simulink subsystem "PvtSubSys_VSM_ESS"  (R2020b)
settings: Solver=VariableStepAuto  StartTime=0.0  StopTime=10.0  RelTol=1e-3
values from neighbouring files (symbols this model uses):
  P_VSM_ESS_AccelPed_enable = 1.0    [ESS.sldd]
  P_VSM_ESS_AccPedlPosn_Param = 60.0    [ESS.sldd]
  P_VSM_ESS_ACtiveTime = 5.0    [ESS.sldd]
  P_VSM_ESS_AEBFlag_enable = 1.0    [ESS.sldd]
  P_VSM_ESS_AngleSpdTable_deg : value not decoded    [ESS.sldd]
  P_VSM_ESS_DangerPlausLeft = 0.3    [ESS.sldd]
  P_VSM_ESS_DangerPlausRight = 0.3    [ESS.sldd]
  P_VSM_ESS_DelayTime = 3.0    [ESS.sldd]
  P_VSM_ESS_DoorSts_enable = 1.0    [ESS.sldd]
  P_VSM_ESS_DriveIn : value not decoded    [ESS.sldd]
  P_VSM_ESS_DriveIn_BP : value not decoded    [ESS.sldd]
  P_VSM_ESS_DriverInputdSameDire_delaytime = 1.0    [ESS.sldd]
  P_VSM_ESS_DriverInputTrq_Param : value not decoded    [ESS.sldd]
  P_VSM_ESS_DrvOverTime_Param = 0.2    [ESS.sldd]
  P_VSM_ESS_DrvOverTime_Paramsame = 0.2    [ESS.sldd]
  P_VSM_ESS_DrvSBR_enable = 1.0    [ESS.sldd]
  P_VSM_ESS_ESPActive_enable = 1.0    [ESS.sldd]
  P_VSM_ESS_ESPFuncOffSts_enable = 1.0    [ESS.sldd]
  P_VSM_ESS_FcwDisFlag_enable = 1.0    [ESS.sldd]
  P_VSM_ESS_FcwSw_enable = 1.0    [ESS.sldd]
  P_VSM_ESS_HiLoBeam_enable = 1.0    [ESS.sldd]
  P_VSM_ESS_IPSpeed_kmh : value not decoded    [ESS.sldd]
  P_VSM_ESS_LateralAccel_enable = 1.0    [ESS.sldd]
  P_VSM_ESS_LgtAccelLower_Param = -8.0    [ESS.sldd]
  P_VSM_ESS_LgtAccelUpper_Param = 3.0    [ESS.sldd]
  P_VSM_ESS_MasterCylindBrake = 5.0    [ESS.sldd]
  P_VSM_ESS_MaxLateral_mss : value not decoded    [ESS.sldd]
  P_VSM_ESS_OVERRIDE_SW = 0.0    [ESS.sldd]
  P_VSM_ESS_SafeDistance_m = 1.5    [ESS.sldd]
  P_VSM_ESS_SpdPoint_kmh : value not decoded    [ESS.sldd]
  P_VSM_ESS_SpdTime_s : value not decoded    [ESS.sldd]
  P_VSM_ESS_SteerWheelSpd_BP : value not decoded    [ESS.sldd]
  P_VSM_ESS_SteerWheelSpd_enable = 1.0    [ESS.sldd]
  P_VSM_ESS_SteerWheelSpd_Param : value not decoded    [ESS.sldd]
  P_VSM_ESS_StopA0_Param = 0.2    [ESS.sldd]
  P_VSM_ESS_StopA1_Param = 0.02    [ESS.sldd]
  P_VSM_ESS_StopA1Time_Param = 2.0    [ESS.sldd]
  P_VSM_ESS_TrailerSts_enable = 1.0    [ESS.sldd]
  P_VSM_ESS_VehLgtAccel_enable = 1.0    [ESS.sldd]
  P_VSM_ESS_Vehspeed_enable = 1.0    [ESS.sldd]
  P_VSM_ESS_WiprReq_enable = 1.0    [ESS.sldd]
undefined symbols (not defined in the file or in its folder): P_Global_WheelBase_m
libraries: simulink x104, TrueDurationTime x6
(part 2 of 3)

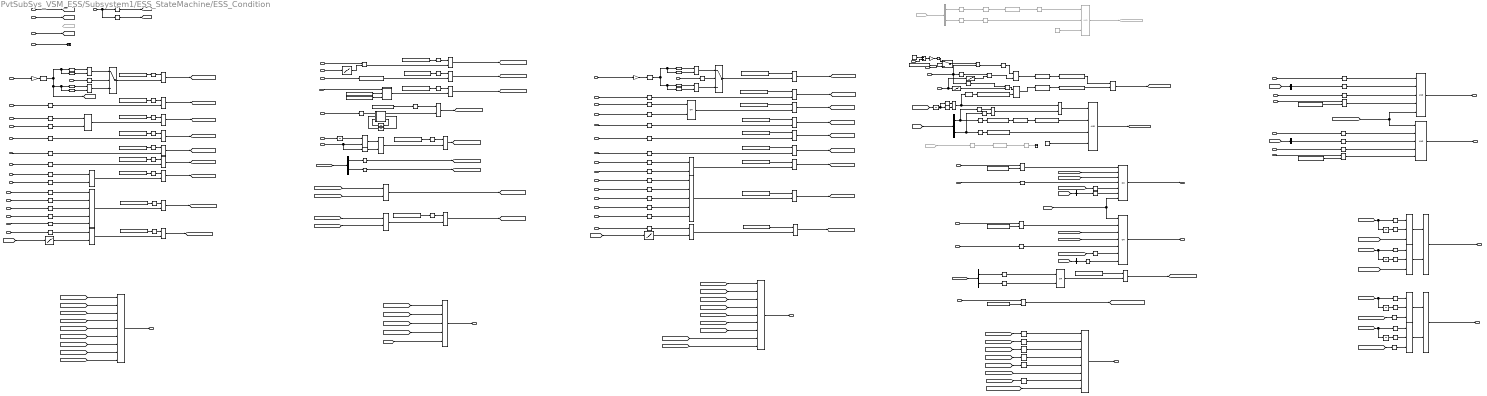
== system PvtSubSys_VSM_ESS/Subsystem1/ESS_StateMachine/ESS_Condition ==
  note: READY2ACYIVE
  note: READY2IDLE
  note: IDLE2READY
  note: PathCondition
  note: EXIT2Ready
  canABSVehicleSpd : Inport
  canESPVDCActive : Inport  Port=2
  canESPPTCActive : Inport  Port=3
  canESPBTCActive : Inport  Port=4
  canABSABSActive : Inport  Port=5
  canEPSEPS_DriverInputTrqValue : Inport  Port=6
  canSASSteerWheelSpd : Inport  Port=7
  canECMAccrPedlPosnDiagc : Inport  Port=8
  canABMLateralAcce : Inport  Port=9
  Torq : Inport  Port=10
  SteerWheelSpdSign : Inport  Port=11
  canBCMWiperSwitchSts : Inport  Port=12
  canBCMHighBeamSts : Inport  Port=13
  canBCMLowBeamSts : Inport  Port=14
  ESPFuncOffSts : Inport  Port=15
  DrvDoorSts : Inport  Port=16
  PassengerDoorSts : Inport  Port=17
  DrvSBR : Inport  Port=18
  canABMLgtAccel : Inport  Port=19
  canESPMSRActive : Inport  Port=20
  canESS_PedSwtReq : Inport  Port=21
  canESP_MasterCylindBrakePress : Inport  Port=22
  TrailerSts : Inport  Port=23
  DangerPlausLeft : Inport  Port=24
  DangerPlausRight : Inport  Port=25
  L_Oncoming_flag : Inport  Port=26
  R_Oncoming_flag : Inport  Port=27
  AEB_Type : Inport  Port=28
  AEBRange : Inport  Port=29
  FCW_Warn : Inport  Port=30
  D_LastPoint : Inport  Port=31
  Target_Line : Inport  Port=32
  ESSState : Inport  Port=33
  AEBTrig : Inport  Port=34
  Dia_inhibit : Inport  Port=35
  steeranglesign : Inport  Port=36
  1-D Lookup Table : Lookup_n-D  NumberOfTableDimensions=1  BreakpointsForDimension1=P_VSM_ESS_IPSpeed_kmh  Table=P_VSM_ESS_MaxLateral_mss  InternalRulePriority=Speed  RndMeth=Simplest  InputSameDT=on
  1-D Lookup Table1 : Lookup_n-D  NumberOfTableDimensions=1  BreakpointsForDimension1=P_VSM_ESS_IPSpeed_kmh  Table=P_VSM_ESS_MaxLateral_mss  InternalRulePriority=Speed  RndMeth=Simplest  InputSameDT=on
  1-D Lookup Table2 : Lookup_n-D  NumberOfTableDimensions=1  BreakpointsForDimension1=P_VSM_ESS_SteerWheelSpd_BP  Table=P_VSM_ESS_SteerWheelSpd_Param  ExtrapMethod=Clip  UseLastTableValue=on  InternalRulePriority=Speed  RndMeth=Simplest  InputSameDT=on
  1-D Lookup Table3 : Lookup_n-D  NumberOfTableDimensions=1  BreakpointsForDimension1=P_VSM_ESS_DriveIn_BP  Table=P_VSM_ESS_DriveIn  InternalRulePriority=Speed  RndMeth=Simplest  InputSameDT=on
  1-D Lookup Table4 : Lookup_n-D  NumberOfTableDimensions=1  BreakpointsForDimension1=P_VSM_ESS_DriveIn_BP  Table=P_VSM_ESS_DriverInputTrq_Param  InternalRulePriority=Speed  RndMeth=Simplest  InputSameDT=on
  ACTIVE2IDLE : Logic  Operator=OR  Inputs=8  AllPortsSameDT=off  OutDataTypeStr=boolean
  Abs{,1,3,16..18} (6 alike) : Abs
  Abs19 : Abs  Commented=on
  Abs2 : Abs  Commented=on
  Add : Sum  Inputs=-+
  Bias4 : Bias  Bias=1.3
  Bias7 : Bias  Bias=1.3
  Bus Selector1 : BusSelector  OutputSignals=ESSLineLValid
  Bus Selector13 : BusSelector  OutputSignals=AEB_PedTrig,AEB_VehTrig
  Bus Selector2 : BusSelector  OutputSignals=AEB_PedTrig,AEB_VehTrig
  Bus Selector20 : BusSelector  OutputSignals=ESSLineA1,ESSLineA0
  Bus Selector21 : BusSelector  Commented=on  OutputSignals=ESSLineA1,ESSLineA0
  Bus Selector3 : BusSelector  OutputSignals=ESSLineLValid
  Bus Selector4 : BusSelector  OutputSignals=ESSLineRValid
  Bus Selector5 : BusSelector  OutputSignals=ESSLineRValid
  Compare To Constant{,11,13,15} (4 alike) : simulink/Logic and Bit Operations/Compare To Constant  relop===  const=2  OutDataTypeStr=boolean
  Compare To Constant1 : simulink/Logic and Bit Operations/Compare To Constant  relop=>=  const=P_VSM_ESS_DrvOverTime_Param  OutDataTypeStr=boolean
  Compare To Constant10 : simulink/Logic and Bit Operations/Compare To Constant  relop===  const=4  OutDataTypeStr=boolean
  Compare To Constant{3,8..9,18,20..32,113,181,184..185,193,195,200..201,214..215,220..224,237} (33 alike) : simulink/Logic and Bit Operations/Compare To Constant  relop===  const=0  OutDataTypeStr=boolean
  Compare To Constant12 : simulink/Logic and Bit Operations/Compare To Constant  relop===  const=5  OutDataTypeStr=boolean
  Compare To Constant14 : simulink/Logic and Bit Operations/Compare To Constant  relop===  const=4  OutDataTypeStr=boolean
  Compare To Constant16 : simulink/Logic and Bit Operations/Compare To Constant  relop===  const=5  OutDataTypeStr=boolean
  Compare To Constant166 : simulink/Logic and Bit Operations/Compare To Constant  relop=>=  const=50  OutDataTypeStr=boolean
  Compare To Constant17 : simulink/Logic and Bit Operations/Compare To Constant  relop=>  const=0  OutDataTypeStr=boolean
  Compare To Constant176 : simulink/Logic and Bit Operations/Compare To Constant  relop=<=  const=100  OutDataTypeStr=boolean
  Compare To Constant179 : simulink/Logic and Bit Operations/Compare To Constant  relop=<=  const=45  OutDataTypeStr=boolean
  Compare To Constant180 : simulink/Logic and Bit Operations/Compare To Constant  relop=>=  const=105  OutDataTypeStr=boolean
  Compare To Constant{6..7,183,188..190,194,196..197,202,205,217..219,226..228,232,235,239..240} (21 alike) : simulink/Logic and Bit Operations/Compare To Constant  relop===  const=1  OutDataTypeStr=boolean
  Compare To Constant19 : simulink/Logic and Bit Operations/Compare To Constant  relop===  const=4  OutDataTypeStr=boolean
  Compare To Constant198 : simulink/Logic and Bit Operations/Compare To Constant  relop=<  const=3  OutDataTypeStr=boolean
  Compare To Constant199 : simulink/Logic and Bit Operations/Compare To Constant  relop===  const=3  OutDataTypeStr=boolean
  Compare To Constant2 : simulink/Logic and Bit Operations/Compare To Constant  relop=>=  const=P_VSM_ESS_StopA1Time_Param  OutDataTypeStr=boolean
  Compare To Constant207 : simulink/Logic and Bit Operations/Compare To Constant  relop=<  const=P_VSM_ESS_AccPedlPosn_Param  OutDataTypeStr=boolean
  Compare To Constant211 : simulink/Logic and Bit Operations/Compare To Constant  relop=<=  const=P_VSM_ESS_StopA1_Param  OutDataTypeStr=boolean
  Compare To Constant212 : simulink/Logic and Bit Operations/Compare To Constant  relop=>  const=0  OutDataTypeStr=boolean
  Compare To Constant216 : simulink/Logic and Bit Operations/Compare To Constant  relop=<=  const=P_VSM_ESS_StopA0_Param  OutDataTypeStr=boolean
  Compare To Constant229 : simulink/Logic and Bit Operations/Compare To Constant  Commented=on  relop=<=  const=0.015  OutDataTypeStr=boolean
  Compare To Constant230 : simulink/Logic and Bit Operations/Compare To Constant  relop=>=  const=50  OutDataTypeStr=boolean
  Compare To Constant231 : simulink/Logic and Bit Operations/Compare To Constant  relop=<=  const=85  OutDataTypeStr=boolean
  Compare To Constant233 : simulink/Logic and Bit Operations/Compare To Constant  relop=<=  const=45  OutDataTypeStr=boolean
  Compare To Constant234 : simulink/Logic and Bit Operations/Compare To Constant  relop=>=  const=90  OutDataTypeStr=boolean
  Compare To Constant236 : simulink/Logic and Bit Operations/Compare To Constant  Commented=on  relop=<=  const=0.2  OutDataTypeStr=boolean
  Compare To Constant33 : simulink/Logic and Bit Operations/Compare To Constant  relop===  const=5  OutDataTypeStr=boolean
  Compare To Constant34 : simulink/Logic and Bit Operations/Compare To Constant  relop=~=  const=0  OutDataTypeStr=boolean
  Compare To Constant35 : simulink/Logic and Bit Operations/Compare To Constant  relop=~=  const=0  OutDataTypeStr=boolean
  Compare To Constant36 : simulink/Logic and Bit Operations/Compare To Constant  relop===  const=3  OutDataTypeStr=boolean
  Compare To Constant37 : simulink/Logic and Bit Operations/Compare To Constant  relop=>=  const=P_VSM_ESS_DriverInputdSameDire_delaytime  OutDataTypeStr=boolean
  Compare To Constant38 : simulink/Logic and Bit Operations/Compare To Constant  relop=>=  const=P_VSM_ESS_DrvOverTime_Paramsame  OutDataTypeStr=boolean
  Compare To Constant4 : simulink/Logic and Bit Operations/Compare To Constant  Commented=on  relop=>=  const=2  OutDataTypeStr=boolean
  Compare To Constant5 : simulink/Logic and Bit Operations/Compare To Constant  Commented=on  relop=>=  const=5  OutDataTypeStr=boolean
  Compare To Zero{,1..5} (6 alike) : simulink/Logic and Bit Operations/Compare To Zero  relop===  OutDataTypeStr=boolean
  Compare To Zero6 : simulink/Logic and Bit Operations/Compare To Zero  relop=<  OutDataTypeStr=boolean
  Compare To Zero7 : simulink/Logic and Bit Operations/Compare To Zero  Commented=on  relop===  OutDataTypeStr=boolean
  Constant : Constant  Value=P_VSM_ESS_DangerPlausLeft
  Constant1 : Constant  Value=P_VSM_ESS_FcwSw_enable
  Constant11 : Constant  OutDataTypeStr=boolean
  Constant12 : Constant  Commented=on  OutDataTypeStr=boolean
  Constant2 : Constant  Value=P_VSM_ESS_MasterCylindBrake
  Constant3 : Constant  Value=P_VSM_ESS_OVERRIDE_SW
  Constant4 : Constant  Value=P_VSM_ESS_DangerPlausRight
  Constant5 : Constant  Value=0.5
  Constant6 : Constant  Value=P_VSM_ESS_DangerPlausLeft
  Constant7 : Constant  Value=P_VSM_ESS_DangerPlausRight
  DangerPlausLeft_1 : InportShadow  Port=24
  DangerPlausRight_1 : InportShadow  Port=25
  DrvDoorSts_1 : InportShadow  Port=16
  DrvSBR_1 : InportShadow  Port=18
  ESPFuncOffSts_1 : InportShadow  Port=15
  ESS_AEBFlag : Logic  AllPortsSameDT=off  OutDataTypeStr=boolean
  ESS_AEBFlag1 : Logic  AllPortsSameDT=off  OutDataTypeStr=boolean
  ESS_AEBFlag2 : Logic  AllPortsSameDT=off  OutDataTypeStr=boolean
  ESS_AEBFlag3 : Logic  Operator=OR  AllPortsSameDT=off  OutDataTypeStr=boolean
  ESS_AEBFlag4 : Logic  Operator=OR  AllPortsSameDT=off  OutDataTypeStr=boolean
  ESS_AEBFlag5 : Logic  Operator=OR  AllPortsSameDT=off  OutDataTypeStr=boolean
  From314 : From  Commented=on  GotoTag=Target_Line
  From316 : From  Commented=on  GotoTag=FCWObjExist
  Gain : Gain  Gain=-2
  Gain15 : Gain  Gain=1.03
  Gain16 : Gain  Gain=1.03
  Goto169 : Goto  Commented=on  GotoTag=ESS_R_Acomp_Active2Ready
  Goto3 : Goto  Commented=on  GotoTag=FCWObjExist
  IDLE2READY : Logic  Inputs=9  AllPortsSameDT=off  OutDataTypeStr=boolean
  L_Oncoming_flag_1 : InportShadow  Port=26
  Logical Operator{,3,6,8..18,28,32,64,103,111,114,128} (21 alike) : Logic  Operator=OR  AllPortsSameDT=off  OutDataTypeStr=boolean
  Logical Operator{1..2,4..5} (4 alike) : Logic  Inputs=3  AllPortsSameDT=off  OutDataTypeStr=boolean
  Logical Operator104 : Logic  Operator=OR  Inputs=7  AllPortsSameDT=off  OutDataTypeStr=boolean
  Logical Operator{7,19..27,29..31,108,110,112..113,127} (18 alike) : Logic  AllPortsSameDT=off  OutDataTypeStr=boolean
  Logical Operator109 : Logic  Operator=OR  Inputs=7  AllPortsSameDT=off  OutDataTypeStr=boolean
  Logical Operator123 : Logic  Inputs=5  AllPortsSameDT=off  OutDataTypeStr=boolean
  Logical Operator125 : Logic  Operator=OR  Inputs=5  AllPortsSameDT=off  OutDataTypeStr=boolean
  Logical Operator45 : Logic  Inputs=5  AllPortsSameDT=off  OutDataTypeStr=boolean
  Logical Operator68 : Logic  Inputs=4  AllPortsSameDT=off  OutDataTypeStr=boolean
  Logical Operator78 : Logic  Inputs=5  AllPortsSameDT=off  OutDataTypeStr=boolean
  Logical Operator81 : Logic  Commented=on  Inputs=3  AllPortsSameDT=off  OutDataTypeStr=boolean
  MATLAB Function : MATLAB Function  TreatAsAtomicUnit=on
  MATLAB Function1 : MATLAB Function  TreatAsAtomicUnit=on
  PassengerDoorSts_1 : InportShadow  Port=17
  Product7 : Product
  READY2ACTIVE : Logic  Inputs=5  AllPortsSameDT=off  OutDataTypeStr=boolean
  READY2IDLE : Logic  Operator=OR  Inputs=9  AllPortsSameDT=off  OutDataTypeStr=boolean
  R_Oncoming_flag_1 : InportShadow  Port=27
  Relational Operator : RelationalOperator  Operator=<=  OutDataTypeStr=boolean  RndMeth=Simplest
  Relational Operator1 : RelationalOperator  Operator=<=  OutDataTypeStr=boolean  RndMeth=Simplest
  Relational Operator13 : RelationalOperator  OutDataTypeStr=boolean  RndMeth=Nearest
  Relational Operator{2..3,5..9} (7 alike) : RelationalOperator  Operator=>  OutDataTypeStr=boolean  RndMeth=Simplest
  Relational Operator4 : RelationalOperator  Operator=<  OutDataTypeStr=boolean  RndMeth=Simplest
  Sign : Signum
  Signal Copy{1..6} (6 alike) : SignalConversion  OverrideOpt=off
  SteerWheelSpdSign_1 : InportShadow  Port=11
  Switch : Switch  Criteria=u2 > Threshold
  Switch10 : Switch  Criteria=u2 ~= 0
  Switch11 : Switch  Criteria=u2 ~= 0
  Terminator : Terminator
  Terminator10 : Terminator
  TrailerSts_1 : InportShadow  Port=23
  TrueDurationTime{,1,4..5} (4 alike) : TrueDurationTime/TrueDurationTime  TCycle=0.02
  TrueDurationTime2 : TrueDurationTime/TrueDurationTime  Commented=on  TCycle=0.02
  TrueDurationTime3 : TrueDurationTime/TrueDurationTime  Commented=on  TCycle=0.02
  Unit Delay{,1..7} (8 alike) : UnitDelay  SampleTime=-1  HasFrameUpgradeWarning=on
  canABMLateralAcce_1 : InportShadow  Port=9
  canABSABSActive_1 : InportShadow  Port=5
  canABSVehicleSpd1 : InportShadow
  canABSVehicleSpd_1 : InportShadow
  canABSVehicleSpd_2 : InportShadow
  canBCMHighBeamSts_1 : InportShadow  Port=13
  canBCMLowBeamSts_1 : InportShadow  Port=14
  canBCMWiperSwitchSts_1 : InportShadow  Port=12
  canESPBTCActive_1 : InportShadow  Port=4
  canESPMSRActive_1 : InportShadow  Port=20
  canESPPTCActive_1 : InportShadow  Port=3
  canESPVDCActive_1 : InportShadow  Port=2
  canESS_PedSwtReq_1 : InportShadow  Port=21
  param_1 : Constant  Value=P_VSM_ESS_Vehspeed_enable
  param_10 : Constant  Value=P_VSM_ESS_SteerWheelSpd_enable
  param_11 : Constant  Value=P_VSM_ESS_AccelPed_enable
  param_12 : Constant  Value=P_VSM_ESS_VehLgtAccel_enable
  param_13 : Constant  Value=P_VSM_ESS_FcwDisFlag_enable
  param_14 : Constant  Value=P_VSM_ESS_AEBFlag_enable
  param_15 : Constant  Value=P_VSM_ESS_ESPFuncOffSts_enable
  param_16 : Constant  Value=P_VSM_ESS_DoorSts_enable
  param_17 : Constant  Value=P_VSM_ESS_DrvSBR_enable
  param_18 : Constant  Value=P_VSM_ESS_TrailerSts_enable
  param_19 : Constant  Value=P_VSM_ESS_WiprReq_enable
  param_2 : Constant  Value=P_VSM_ESS_ESPFuncOffSts_enable
  param_20 : Constant  Value=P_VSM_ESS_HiLoBeam_enable
  param_21 : Constant  Value=P_VSM_ESS_ESPActive_enable
  param_22 : Constant  Value=P_VSM_ESS_LateralAccel_enable
  param_23 : Constant  Value=P_VSM_ESS_AEBFlag_enable
  param_24 : Constant  Value=P_VSM_ESS_LgtAccelUpper_Param
  param_25 : Constant  Value=P_VSM_ESS_LgtAccelLower_Param
  param_3 : Constant  Value=P_VSM_ESS_DoorSts_enable
  param_4 : Constant  Value=P_VSM_ESS_DrvSBR_enable
  param_5 : Constant  Value=P_VSM_ESS_TrailerSts_enable
  param_52 : Constant  Value=P_VSM_ESS_Vehspeed_enable
  param_6 : Constant  Value=P_VSM_ESS_WiprReq_enable
  param_7 : Constant  Value=P_VSM_ESS_HiLoBeam_enable
  param_8 : Constant  Value=P_VSM_ESS_ESPActive_enable
  param_9 : Constant  Value=P_VSM_ESS_LateralAccel_enable
  ESSDataClct_DriverSteerESSExit : Outport
  ESSDataClct_OverrideESSExit : Outport  Port=2
  ESS_IDLE2READY : Outport  Port=3
  ESS_READY2ACTIVE : Outport  Port=4
  ESS_READY2IDLE : Outport  Port=5
  ESS_ACTIVE2IDLE : Outport  Port=6
  ESS_L_Active2Ready : Outport  Port=7
  ESS_R_Active2Ready : Outport  Port=8
  ESS_Left_Ready2Active : Outport  Port=9
  ESS_Right_Ready2Active : Outport  Port=10
  wires:
  Abs3/1 -> Relational Operator9/1
  1-D Lookup Table4/1 -> Relational Operator9/2
  Logical Operator32/1 -> [ESS_DrvOver_Active2Ready]  "VSM_ESS_DrvOver_Active2Ready"
  Compare To Constant38/1 -> Logical Operator32/2  "VSM_ESS_DrvOver_Active2Ready_SamDirc"
  TrueDurationTime5/1 -> Compare To Constant38/1
  Logical Operator31/1 -> TrueDurationTime5/1
  Relational Operator8/1 -> Logical Operator31/1
  Compare To Constant37/1 -> Logical Operator31/2
  TrueDurationTime4/1 -> Compare To Constant37/1
  1-D Lookup Table3/1 -> Relational Operator8/2
  Abs/1 -> Relational Operator8/1
  canABSVehicleSpd_2/1 -> 1-D Lookup Table3/1, 1-D Lookup Table4/1
  Sign/1 -> Switch/1
  1-D Lookup Table2/1 -> Relational Operator7/2
  canABSVehicleSpd1/1 -> 1-D Lookup Table2/1
  [Dia_Out] -> Logical Operator104/1, Logical Operator109/7
  [Dia_In] -> READY2ACTIVE/5
  Compare To Constant36/1 -> [Dia_Out]
  Compare To Constant3/1 -> [Dia_In]
  Dia_inhibit/1 -> Compare To Constant3/1, Compare To Constant36/1
  param_25/1 -> MATLAB Function1/3(lower)
  param_24/1 -> MATLAB Function1/2(uper)
  DangerPlausRight_1/1 -> Relational Operator1/1
  Signal Copy5/1 -> ACTIVE2IDLE/5  "VSM_ESS_DrvSBR_ACTIVE2IDLE"
  Compare To Constant16/1 -> Logical Operator5/2
  Compare To Constant211/1 -> TrueDurationTime1/1
  Logical Operator9/1 -> [Con_DoorSts_Idle2Ready_ESS]  "VSM_ESS_DoorSts_IDLE2READY"
  Compare To Constant216/1 -> Logical Operator68/3  "VSM_ESS_LineA0_Active2Ready"
  Logical Operator104/1 -> ESS_R_Active2Ready/1  "VSM_ESS_R_Active2Ready"
  canSASSteerWheelSpd/1 -> Relational Operator7/1
  [Con_HiLoBeam_Ready2Idle_ESS] -> READY2IDLE/7
  Unit Delay5/1 -> Compare To Constant16/1
  [Con_AccelPedl_Ready2Active_ESS] -> READY2ACTIVE/3
  [Con_AEBFlag_Ready2Active_ESS] -> READY2ACTIVE/2
  [Con_FcwFlag_Ready2Active_ESS] -> READY2ACTIVE/1
  Bias4/1 -> Compare To Constant230/1, Compare To Constant231/1, [IP_Speed], Compare To Constant176/1, Compare To Constant166/1
  [Con_HiLoBeam_Idle2Ready_ESS] -> IDLE2READY/7
  Logical Operator1/1 -> Logical Operator3/1
  canESPMSRActive/1 -> Compare To Constant221/1
  [Con_WiprReq_Ready2Idle_ESS] -> READY2IDLE/6
  Signal Copy3/1 -> ACTIVE2IDLE/4  "VSM_ESS_DoorSts_ACTIVE2IDLE"
  Compare To Constant179/1 -> Logical Operator128/1
  DrvDoorSts/1 -> Compare To Constant184/1
  [Con_DoorSts_Idle2Ready_ESS] -> IDLE2READY/3
  Compare To Constant231/1 -> Logical Operator127/2
  [Con_VehLgtAccel_Ready2Active_ESS] -> READY2ACTIVE/4
  Bus Selector4/1 -> Compare To Constant196/1  "<ESSLineRValid>"
  canABSABSActive_1/1 -> Compare To Constant227/1
  Compare To Zero/1 -> Logical Operator45/3  "VSM_ESS_LeftOncoming_Ready2Active"
  Compare To Constant226/1 -> Logical Operator125/3
  Logical Operator108/1 -> TrueDurationTime/1
  ESS_AEBFlag1/1 -> [Con_FcwFlag_Ready2Active_ESS]  "VSM_ESS_FcwFlag_READY2ACTIVE"
  SteerWheelSpdSign_1/1 -> Compare To Constant217/1
  Compare To Constant180/1 -> Logical Operator128/2
  [Con_ESPFuncOffSts_Ready2Idle_ESS] -> READY2IDLE/2
  Compare To Constant227/1 -> Logical Operator125/5
  [Con_DrvSBR_Idle2Ready_ESS] -> IDLE2READY/4
  Signal Copy1/1 -> ACTIVE2IDLE/2  "VSM_ESS_LateralAccel_ACTIVE2IDLE"
  [Con_VehicleSpeed_Idle2Ready_ESS] -> IDLE2READY/1
  Bus Selector13/1 -> Compare To Constant214/1  "<AEB_PedTrig>"
  Abs17/1 -> Relational Operator5/1
  [Target_Line] -> Bus Selector5/1
  canESPPTCActive/1 -> Compare To Constant223/1
  R_Oncoming_flag_1/1 -> Compare To Zero3/1
  [Con_TrailerSts_Idle2Ready_ESS] -> IDLE2READY/5
  canESPBTCActive/1 -> Compare To Constant224/1
  [Target_Line] -> Bus Selector1/1
  [Con_TrailerSts_Ready2Idle_ESS] -> READY2IDLE/5
  Logical Operator6/1 -> ESSDataClct_OverrideESSExit/1  "ESSDataClct_OverrideESSExit"
  Compare To Zero4/1 -> Logical Operator4/3
  [Con_VehicleSpeed_Ready2Idle_ESS] -> READY2IDLE/1
  canESPVDCActive/1 -> Compare To Constant222/1
  [Con_ABMLateralAcce_Idle2Ready_ESS] -> IDLE2READY/9
  Logical Operator18/1 -> [Con_VehLgtAccel_Ready2Active_ESS]  "VSM_ESS_VehLgtAccel_READY2ACTIVE"
  Compare To Constant219/1 -> Logical Operator125/2
  Constant11/1 -> Logical Operator68/4
  Bias7/1 -> Compare To Constant233/1, Compare To Constant234/1, Compare To Constant180/1, Compare To Constant179/1
  Compare To Constant166/1 -> Logical Operator110/1
  [ESS_Acomp_Active2Ready] -> Logical Operator104/3
  DrvSBR_1/1 -> Compare To Constant194/1
  ESS_AEBFlag5/1 -> [Con_AEBFlag_Ready2Active_ESS]  "VSM_ESS_AEBFlag_READY2ACTIVE"
  PassengerDoorSts/1 -> Compare To Constant185/1
  PassengerDoorSts_1/1 -> Compare To Constant189/1
  Logical Operator21/1 -> [Con_DrvSBR_Ready2Idle_ESS]  "VSM_ESS_DrvSBR_READY2IDLE"
  [Con_DrvSBR_Ready2Idle_ESS] -> READY2IDLE/4
  Signal Copy2/1 -> ACTIVE2IDLE/3  "VSM_ESS_ESPFuncOffSts_ACTIVE2IDLE"
  ESPFuncOffSts/1 -> Compare To Constant181/1
  [Con_WiprReq_Idle2Ready_ESS] -> IDLE2READY/6
  Compare To Constant190/1 -> Logical Operator45/2  "VSM_ESS_LineLValid_Ready2Active"
  Logical Operator127/1 -> Switch10/1
  canABMLgtAccel/1 -> MATLAB Function1/1(LgAcc)
  IDLE2READY/1 -> ESS_IDLE2READY/1
  Compare To Constant237/1 -> Logical Operator45/1  "VSM_ESS_L_SteerWheelSpdSign_Ready2Active"
  Logical Operator7/1 -> [Con_VehicleSpeed_Ready2Idle_ESS]  "VSM_ESS_VehicleSpd_READY2IDLE"
  Logical Operator64/1 -> [Con_VehicleSpeed_Idle2Ready_ESS]  "VSM_ESS_VehicleSpd_IDLE2READY"
  Bus Selector13/2 -> Compare To Constant215/1  "<AEB_VehTrig>"
  [Con_ESPFuncOffSts_Idle2Ready_ESS] -> IDLE2READY/2
  DrvSBR/1 -> Compare To Constant193/1
  ESPFuncOffSts_1/1 -> Compare To Constant183/1
  canESPBTCActive_1/1 -> Compare To Constant228/1
  canBCMHighBeamSts/1 -> Compare To Constant200/1
  TrueDurationTime1/1 -> Compare To Constant2/1
  Abs19/1 -> Compare To Constant229/1
  Logical Operator78/1 -> ESS_Right_Ready2Active/1
  Compare To Constant189/1 -> Logical Operator103/2
  L_Oncoming_flag/1 -> Compare To Constant239/1
  AEBRange/1 -> Unit Delay/1
  Compare To Constant215/1 -> [Con_AEBVehFlag_Ready2Active_ESS]
  TrailerSts_1/1 -> Compare To Constant197/1
  Logical Operator26/1 -> [Con_ABMLateralAcce_Ready2Idle_ESS]  "VSM_ESS_LateralAccel_READY2IDLE"
  [ESSState] -> Unit Delay1/1, Compare To Constant/1
  Compare To Constant240/1 -> Logical Operator104/5  "VSM_ESS_R_Oncoming_Active2Ready"
  DangerPlausLeft/1 -> Relational Operator2/1
  Logical Operator15/1 -> [Con_ABMLateralAcce_Idle2Ready_ESS]  "VSM_ESS_LateralAccel_IDLE2READY"
  Logical Operator11/1 -> [Con_TrailerSts_Idle2Ready_ESS]  "VSM_ESS_TrailerSts_IDLE2READY"
  Compare To Constant222/1 -> Logical Operator123/3
  D_LastPoint/1 -> Compare To Constant17/1, Relational Operator13/2
  Compare To Constant13/1 -> Logical Operator4/1
  Compare To Constant11/1 -> Logical Operator2/1
  Abs16/1 -> Relational Operator4/1
  READY2ACTIVE/1 -> ESS_READY2ACTIVE/1
  [Con_AEBVehFlag_Ready2Active_ESS] -> ESS_AEBFlag/1  "VSM_ESS_AEBVehFlag_Ready2Active"
  Logical Operator25/1 -> [Con_ESPActive_Ready2Idle_ESS]  "VSM_ESS_ESPActive_READY2IDLE"
  ESS_AEBFlag2/1 -> ESS_AEBFlag4/2
  DrvDoorSts_1/1 -> Compare To Constant188/1
  Compare To Constant196/1 -> Logical Operator78/3  "VSM_ESS_LineRValid_Ready2Active"
  canABMLateralAcce/1 -> Abs16/1
  Logical Operator20/1 -> [Con_DoorSts_Ready2Idle_ESS]  "VSM_ESS_DoorSts_READY2IDLE"
  Unit Delay4/1 -> Compare To Constant14/1
  Logical Operator109/1 -> ESS_L_Active2Ready/1  "VSM_ESS_L_Active2Ready"
  Compare To Constant4/1 -> Logical Operator81/1  "VSM_ESS_LineRA1_Active2Ready"
  Bus Selector21/2 -> Abs2/1  "<ESSLineA0>"
  Unit Delay2/1 -> Compare To Constant12/1
  Compare To Constant202/1 -> Logical Operator114/1
  [ESS_DrvOver_Active2Ready] -> Logical Operator104/4
  Relational Operator1/1 -> Logical Operator78/5  "VSM_ESS_DangerPlausRight_Ready2Active"
  Logical Operator68/1 -> [ESS_Acomp_Active2Ready]
  [AEBTrig] -> Bus Selector13/1
  Logical Operator16/1 -> [Con_SteerWheelSpd_Ready2Active_ESS]  "VSM_ESS_SteerWheelSpd_READY2ACTIVE"
  Compare To Constant239/1 -> Logical Operator109/4  "VSM_ESS_L_Oncoming_Active2Ready"
  Relational Operator9/1 -> Logical Operator108/2
  Relational Operator3/1 -> Logical Operator104/2  "VSM_ESS_DPC_R_Active2Ready"
  [Target_Line] -> Bus Selector4/1
  canESS_PedSwtReq_1/1 -> Compare To Constant232/1
  Compare To Zero1/1 -> Logical Operator109/5
  Logical Operator128/1 -> Switch11/3
  [ESSState] -> Unit Delay4/1, Compare To Constant13/1
  L_Oncoming_flag_1/1 -> Compare To Zero/1
  Logical Operator14/1 -> [Con_ESPActive_Idle2Ready_ESS]  "VSM_ESS_ESPActive_IDLE2READY"
  FCW_Warn/1 -> Compare To Constant212/1
  Logical Operator81/1 -> Goto169/1
  Compare To Constant15/1 -> Logical Operator5/1
  Compare To Constant184/1 -> Logical Operator113/1
  AEB_Type/1 -> Terminator/1
  Logical Operator17/1 -> [Con_AccelPedl_Ready2Active_ESS]  "VSM_ESS_AccelPed_READY2ACTIVE"
  Abs2/1 -> Compare To Constant236/1
  Compare To Constant200/1 -> Logical Operator112/1
  Compare To Constant217/1 -> Logical Operator78/2  "VSM_ESS_R_SteerWheelSpdSign_Ready2Active"
  canBCMLowBeamSts/1 -> Compare To Constant201/1
  Compare To Constant5/1 -> Terminator10/1
  Gain15/1 -> Bias4/1
  Compare To Constant223/1 -> Logical Operator123/4
  Compare To Constant188/1 -> Logical Operator103/1
  canBCMLowBeamSts_1/1 -> Compare To Constant205/1
  canABSABSActive/1 -> Compare To Constant220/1
  canEPSEPS_DriverInputTrqValue/1 -> Product7/2, Abs3/1, Abs/1
  Logical Operator23/1 -> [Con_WiprReq_Ready2Idle_ESS]  "VSM_ESS_WiprReq_READY2IDLE"
  Gain16/1 -> Bias7/1
  Product7/1 -> Compare To Zero6/1
  [ESS_DrvOver_Active2Ready] -> Logical Operator2/3
  Logical Operator45/1 -> ESS_Left_Ready2Active/1
  canABMLateralAcce_1/1 -> Abs17/1
  [Con_AEBTrigFlag_Active2Idle_ESS] -> ACTIVE2IDLE/6
  Bus Selector21/1 -> Abs19/1  "<ESSLineA1>"
  Compare To Constant185/1 -> Logical Operator113/2
  Compare To Constant236/1 -> Logical Operator81/2  "VSM_ESS_LineRA0_Active2Ready"
  Compare To Constant1/1 -> Logical Operator32/1  "VSM_ESS_DrvOver_Active2Ready_DiffDirc"
  Bus Selector20/1 -> Compare To Constant34/1, Abs18/1  "<ESSLineA1>"
  Compare To Constant235/1 -> Switch11/2
  Abs18/1 -> Compare To Constant211/1
  [Con_AEBVruFlag_Ready2Active_ESS] -> ESS_AEBFlag/2  "VSM_ESS_AEBVruFlag_Ready2Active"
  TrailerSts/1 -> Compare To Constant195/1
  Compare To Constant234/1 -> Logical Operator111/2
  canESPVDCActive_1/1 -> Compare To Constant219/1
  canABSVehicleSpd_1/1 -> Gain16/1
  Compare To Constant/1 -> Logical Operator1/1
  [ESS_Acomp_Active2Ready] -> Logical Operator109/2
  [Con_ESPActive_Idle2Ready_ESS] -> IDLE2READY/8
  Compare To Constant233/1 -> Logical Operator111/1
  Bus Selector2/1 -> Compare To Constant6/1  "<AEB_PedTrig>"
  Compare To Constant232/1 -> Switch10/2
  Logical Operator24/1 -> [Con_HiLoBeam_Ready2Idle_ESS]  "VSM_ESS_HiLoBeam_READY2IDLE"
  [ESS_DrvOver_Active2Ready] -> Logical Operator109/3
  [Target_Line] -> Bus Selector20/1
  Bus Selector1/1 -> Compare To Constant190/1  "<ESSLineLValid>"
  Bus Selector2/2 -> Compare To Constant7/1  "<AEB_VehTrig>"
  DangerPlausRight/1 -> Relational Operator3/1
  Compare To Constant218/1 -> Logical Operator125/1
  TrueDurationTime2/1 -> Compare To Constant5/1
  Compare To Zero7/1 -> TrueDurationTime2/1
  Logical Operator19/1 -> [Con_ESPFuncOffSts_Ready2Idle_ESS]  "VSM_ESS_ESPFuncOffSts_READY2IDLE"
  Logical Operator12/1 -> [Con_WiprReq_Idle2Ready_ESS]  "VSM_ESS_WiprReq_IDLE2READY"
  Logical Operator8/1 -> [Con_ESPFuncOffSts_Idle2Ready_ESS]  "VSM_ESS_ESPFuncOffSts_IDLE2READY"
  TrueDurationTime3/1 -> Compare To Constant4/1
  Compare To Constant229/1 -> TrueDurationTime3/1
  From314/1 -> Bus Selector21/1
  Abs1/1 -> Compare To Constant216/1
  Compare To Zero5/1 -> Logical Operator5/3
  Compare To Constant230/1 -> Logical Operator127/1
  Logical Operator110/1 -> Switch10/3
  Compare To Zero2/1 -> Logical Operator104/6
  canBCMHighBeamSts_1/1 -> Compare To Constant202/1
  Compare To Constant7/1 -> Logical Operator/2
  canESS_PedSwtReq/1 -> Compare To Constant235/1
  Compare To Constant205/1 -> Logical Operator114/2
  Compare To Constant2/1 -> Logical Operator68/2  "VSM_ESS_LineA1_Active2Ready"
  Compare To Constant224/1 -> Logical Operator123/5
  [Con_FcwWarn_Ready2Active_ESS] -> ESS_AEBFlag1/1  "VSM_ESS_FcwWarn_Ready2Active"
  [Con_ABMLateralAcce_Ready2Idle_ESS] -> READY2IDLE/9
  Compare To Constant212/1 -> MATLAB Function/1(u)
  [Con_AccelPedl_Ready2Active_ESS] -> Compare To Zero4/1
  Bus Selector3/1 -> Compare To Constant8/1  "<ESSLineLValid>"
  Signal Copy4/1 -> ACTIVE2IDLE/1  "VSM_ESS_ESPActive_ACTIVE2IDLE"
  [Con_FcwDisFlag_Ready2Active_ESS] -> ESS_AEBFlag1/2  "VSM_ESS_FcwDisFlag_Ready2Active"
  [Target_Line] -> Bus Selector3/1
  [ESSState] -> Compare To Constant11/1, Unit Delay2/1
  [Con_DoorSts_Ready2Idle_ESS] -> READY2IDLE/3
  Logical Operator22/1 -> [Con_TrailerSts_Ready2Idle_ESS]  "VSM_ESS_TrailerSts_READY2IDLE"
  [Con_AccelPedl_Ready2Active_ESS] -> Compare To Zero2/1
  Compare To Constant214/1 -> [Con_AEBVruFlag_Ready2Active_ESS]
  DangerPlausLeft_1/1 -> Relational Operator/1
  Bus Selector5/1 -> Compare To Constant9/1  "<ESSLineRValid>"
  canBCMWiperSwitchSts/1 -> Compare To Constant198/1
  Compare To Zero6/1 -> Logical Operator108/1
  Relational Operator/1 -> Logical Operator45/4  "VSM_ESS_DangerPlausLeft_Ready2Active"
  Compare To Constant8/1 -> Logical Operator109/6  "VSM_ESS_LValid_Active2Ready"
  Compare To Constant12/1 -> Logical Operator2/2
  Logical Operator2/1 -> Logical Operator3/2
  Unit Delay1/1 -> Compare To Constant10/1
  SteerWheelSpdSign/1 -> Compare To Constant237/1
  canABSVehicleSpd/1 -> Gain15/1
  From316/1 -> Compare To Zero7/1
  ACTIVE2IDLE/1 -> ESS_ACTIVE2IDLE/1
  Compare To Zero3/1 -> Logical Operator78/4  "VSM_ESS_RightOncoming_Ready2Active"
  R_Oncoming_flag/1 -> Compare To Constant240/1
  Logical Operator3/1 -> ESSDataClct_DriverSteerESSExit/1  "ESSDataClct_DriverSteerESSExit"
  TrueDurationTime/1 -> Compare To Constant1/1
  Bus Selector20/2 -> Compare To Constant35/1, Abs1/1  "<ESSLineA0>"
  Compare To Constant176/1 -> Logical Operator110/2
  [Con_AccelPedl_Ready2Active_ESS] -> Compare To Zero1/1
  Compare To Constant221/1 -> Logical Operator123/2
  Compare To Constant6/1 -> Logical Operator/1
  READY2IDLE/1 -> ESS_READY2IDLE/1
  [AEBTrig] -> Bus Selector2/1
  Constant12/1 -> Logical Operator81/3
  Compare To Constant10/1 -> Logical Operator1/2
  Compare To Constant14/1 -> Logical Operator4/2
  [Con_ESPActive_Ready2Idle_ESS] -> READY2IDLE/8
  Logical Operator27/1 -> [Con_AEBTrigFlag_Active2Idle_ESS]  "VSM_ESS_AEBTrigFlag_ACTIVE2IDLE"
  Logical Operator111/1 -> Switch11/1
  canESPMSRActive_1/1 -> Compare To Constant218/1
  Logical Operator13/1 -> [Con_HiLoBeam_Idle2Ready_ESS]  "VSM_ESS_HiLoBeam_IDLE2READY"
  canECMAccrPedlPosnDiagc/1 -> Compare To Constant207/1
  [ESSState] -> Compare To Constant15/1, Unit Delay5/1
  Relational Operator2/1 -> Logical Operator109/1  "VSM_ESS_DPC_L_Active2Ready"
  Compare To Constant201/1 -> Logical Operator112/2
  [ESS_DrvOver_Active2Ready] -> Logical Operator1/3
  Logical Operator5/1 -> Logical Operator6/2
  Compare To Constant9/1 -> Logical Operator104/7  "VSM_ESS_RValid_Active2Ready"
  Logical Operator10/1 -> [Con_DrvSBR_Idle2Ready_ESS]  "VSM_ESS_DrvSBR_IDLE2READY"
  Compare To Constant220/1 -> Logical Operator123/1
  Compare To Constant228/1 -> Logical Operator125/4
  Logical Operator4/1 -> Logical Operator6/1
  canESPPTCActive_1/1 -> Compare To Constant226/1
  canBCMWiperSwitchSts_1/1 -> Compare To Constant199/1
  [Con_AccelPedl_Ready2Active_ESS] -> Compare To Zero5/1
  Target_Line/1 -> [Target_Line]
  ESSState/1 -> [ESSState]
  canESP_MasterCylindBrakePress/1 -> Relational Operator6/1
  AEBTrig/1 -> [AEBTrig]
  Relational Operator13/1 -> ESS_AEBFlag2/1
  Compare To Constant17/1 -> ESS_AEBFlag2/2
  Constant/1 -> Relational Operator/2
  Constant4/1 -> Relational Operator1/2
  Constant6/1 -> Relational Operator2/2
  Constant7/1 -> Relational Operator3/2
  [Con_ESPActive_Ready2Idle_ESS] -> Signal Copy4/1
  [Con_ABMLateralAcce_Ready2Idle_ESS] -> Signal Copy1/1
  [Con_ESPFuncOffSts_Ready2Idle_ESS] -> Signal Copy2/1
  [Con_DoorSts_Ready2Idle_ESS] -> Signal Copy3/1
  [Con_DrvSBR_Ready2Idle_ESS] -> Signal Copy5/1
  ESS_AEBFlag3/1 -> [Con_FcwWarn_Ready2Active_ESS]
  Compare To Constant18/1 -> ESS_AEBFlag3/1
  Constant1/1 -> Compare To Constant18/1
  Switch10/1 -> Logical Operator64/2
  Compare To Constant113/1 -> Logical Operator64/1
  param_52/1 -> Compare To Constant113/1
  param_1/1 -> Logical Operator7/1
  Switch11/1 -> Logical Operator7/2
  MATLAB Function/1(y) -> ESS_AEBFlag3/2
  MATLAB Function/2(fg) -> Unit Delay3/1
  Unit Delay3/1 -> MATLAB Function/2(fgk1)
  MATLAB Function/3(c) -> Unit Delay6/1
  Unit Delay6/1 -> MATLAB Function/3(ck1)
  Compare To Constant181/1 -> Logical Operator8/2
  Compare To Constant20/1 -> Logical Operator8/1
  param_2/1 -> Compare To Constant20/1
  Logical Operator113/1 -> Logical Operator9/2
  param_3/1 -> Compare To Constant21/1
  Compare To Constant21/1 -> Logical Operator9/1
  Compare To Constant193/1 -> Logical Operator10/2
  Compare To Constant22/1 -> Logical Operator10/1
  param_4/1 -> Compare To Constant22/1
  Compare To Constant195/1 -> Logical Operator11/2
  param_5/1 -> Compare To Constant23/1
  Compare To Constant23/1 -> Logical Operator11/1
  Compare To Constant198/1 -> Logical Operator12/2
  param_6/1 -> Compare To Constant24/1
  Compare To Constant24/1 -> Logical Operator12/1
  Logical Operator112/1 -> Logical Operator13/2
  param_7/1 -> Compare To Constant25/1
  Compare To Constant25/1 -> Logical Operator13/1
  Logical Operator123/1 -> Logical Operator14/2
  Compare To Constant26/1 -> Logical Operator14/1
  param_8/1 -> Compare To Constant26/1
  param_9/1 -> Compare To Constant27/1
  Compare To Constant27/1 -> Logical Operator15/1
  Relational Operator4/1 -> Logical Operator15/2
  param_10/1 -> Compare To Constant28/1
  Compare To Constant28/1 -> Logical Operator16/1
  Relational Operator7/1 -> Logical Operator16/2
  param_11/1 -> Compare To Constant29/1
  Compare To Constant29/1 -> Logical Operator17/1
  Compare To Constant207/1 -> Logical Operator17/2
  MATLAB Function1/1(y) -> Logical Operator18/2
  param_12/1 -> Compare To Constant30/1
  Compare To Constant30/1 -> Logical Operator18/1
  ESS_AEBFlag4/1 -> [Con_FcwDisFlag_Ready2Active_ESS]
  Compare To Constant31/1 -> ESS_AEBFlag4/1
  param_13/1 -> Compare To Constant31/1
  ESS_AEBFlag/1 -> ESS_AEBFlag5/2
  Compare To Constant32/1 -> ESS_AEBFlag5/1
  param_14/1 -> Compare To Constant32/1
  Compare To Constant183/1 -> Logical Operator19/2
  Logical Operator103/1 -> Logical Operator20/2
  Compare To Constant194/1 -> Logical Operator21/2
  Compare To Constant197/1 -> Logical Operator22/2
  Compare To Constant199/1 -> Logical Operator23/2
  Logical Operator114/1 -> Logical Operator24/2
  Logical Operator125/1 -> Logical Operator25/2
  Relational Operator5/1 -> Logical Operator26/2
  param_15/1 -> Logical Operator19/1
  param_16/1 -> Logical Operator20/1
  param_17/1 -> Logical Operator21/1
  param_18/1 -> Logical Operator22/1
  param_19/1 -> Logical Operator23/1
  param_20/1 -> Logical Operator24/1
  param_21/1 -> Logical Operator25/1
  param_22/1 -> Logical Operator26/1
  Logical Operator/1 -> Logical Operator27/2
  param_23/1 -> Logical Operator27/1
  [IP_Speed] -> 1-D Lookup Table/1
  1-D Lookup Table/1 -> Relational Operator4/2
  1-D Lookup Table1/1 -> Relational Operator5/2
  [IP_Speed] -> 1-D Lookup Table1/1
  Unit Delay7/1 -> Compare To Constant19/1, Compare To Constant33/1
  Logical Operator30/1 -> Logical Operator29/2
  Logical Operator29/1 -> Logical Operator68/1
  Logical Operator28/1 -> Logical Operator29/1, TrueDurationTime4/1
  Compare To Constant19/1 -> Logical Operator28/2
  Compare To Constant33/1 -> Logical Operator28/1
  [ESSState] -> Unit Delay7/1
  Compare To Constant34/1 -> Logical Operator30/1
  Compare To Constant35/1 -> Logical Operator30/2
  [Con_SteerWheelSpd_Ready2Active_ESS] -> Logical Operator78/1, Logical Operator45/5
  Unit Delay/1 -> Relational Operator13/1
  [Con_VehicleSpeed_Ready2Idle_ESS] -> Signal Copy6/1
  Signal Copy6/1 -> ACTIVE2IDLE/7  "VSM_ESS_VehicleSpd_ACTIVE2IDLE"
  Constant2/1 -> Relational Operator6/2
  Relational Operator6/1 -> [Con_MasterCylindBrakePress_Active2Idle_ESS]  "VSM_ESS_MasterCylindBrakePress_ACTIVE2IDLE"
  [Con_MasterCylindBrakePress_Active2Idle_ESS] -> ACTIVE2IDLE/8
  Torq/1 -> Switch/3
  Constant3/1 -> Switch/2
  steeranglesign/1 -> Add/2
  Constant5/1 -> Add/1
  Add/1 -> Gain/1
  Gain/1 -> Sign/1
  Switch/1 -> Product7/1
